simulink model "CenterOfPressure_Integration_TestModel"  (R2014a)
settings: Solver=ode45  StartTime=0.0  StopTime=10.0  RelTol=1e-3
InitFcn:
  | %fins_count=3
  | %height_fins=0.095
  | %fin_center_distance=0.15
  | %fin_tip_chord=0.1
  | %fin_root_chord=0.35
  | %diameter_outer=0.103
  | %d_nose_tip_to_fins=1
  | %height_nose_cone=0.5
  | data_parametric_model
libraries: rocket_angular_flight_library x3
settings Model: Creator=scorpii  LastModifiedBy=scorpii

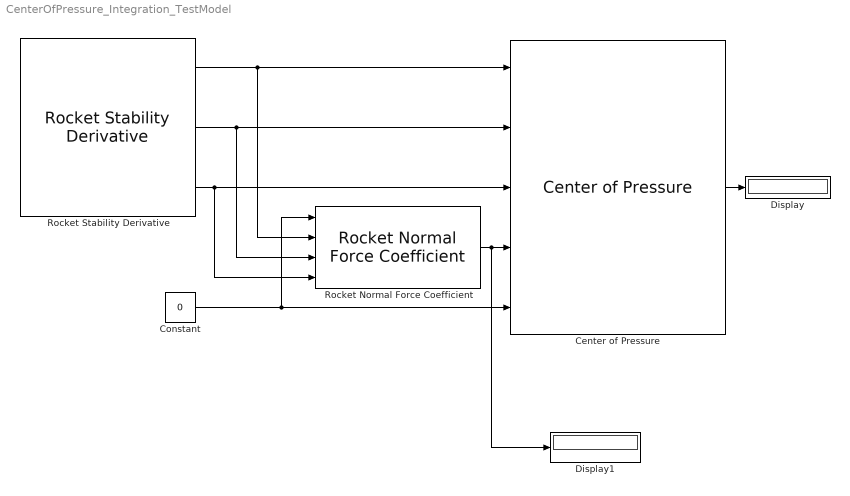
== system CenterOfPressure_Integration_TestModel ==
  Center of Pressure : rocket_angular_flight_library/Center of Pressure
  Constant : Constant  Value=0
  Display : Display
  Display1 : Display
  Rocket Normal Force Coefficient : rocket_angular_flight_library/Rocket Normal Force Coefficient
  Rocket Stability Derivative : rocket_angular_flight_library/Rocket Stability Derivative
  wires:
  Rocket Stability Derivative/2 -> Rocket Normal Force Coefficient/3, Center of Pressure/2
  Rocket Stability Derivative/1 -> Rocket Normal Force Coefficient/2, Center of Pressure/1
  Rocket Stability Derivative/3 -> Center of Pressure/3, Rocket Normal Force Coefficient/4
  Rocket Normal Force Coefficient/1 -> Display1/1, Center of Pressure/4
  Constant/1 -> Rocket Normal Force Coefficient/1, Center of Pressure/5
  Center of Pressure/1 -> Display/1
